simulink model "c3"  (R2019b)
settings: Solver=VariableStepAuto  StartTime=0.0  StopTime=10.0  RelTol=1e-3
values from neighbouring files (symbols this model uses):
  a1 = 1.2    [setup.m]
  a2 = -0.9    [setup.m]
  a3 = 0.25    [setup.m]
  a4 = -0.5    [setup.m]
settings Model: Creator=marcel  LastModifiedBy=marcel

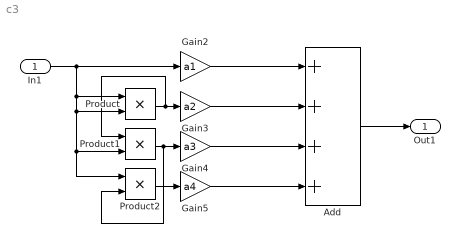
== system c3 ==
  In1 : Inport
  Add : Sum  Inputs=++++
  Gain2 : Gain  Gain=a1
  Gain3 : Gain  Gain=a2
  Gain4 : Gain  Gain=a3
  Gain5 : Gain  Gain=a4
  Product : Product
  Product1 : Product
  Product2 : Product
  Out1 : Outport
  wires:
  Product/1 -> Product1/1, Gain3/1
  In1/1 -> Product2/1, Product1/2, Product/2, Product/1, Gain2/1
  Product2/1 -> Gain5/1
  Product1/1 -> Product2/2, Gain4/1
  Gain2/1 -> Add/1
  Gain4/1 -> Add/3
  Gain3/1 -> Add/2
  Gain5/1 -> Add/4
  Add/1 -> Out1/1
